simulink model "sldemo_eml_galaxy"  (Simulink 6.0)
settings: Solver=FixedStepDiscrete  StartTime=0.0  StopTime=500  FixedStep=1  RelTol=1e-3
settings Model: Creator=The MathWorks Inc.  LastModifiedBy=batserve  ExtModeAutoUpdateStatusClock=off
settings DebuggingCC: CheckExecutionContextPreStartOutputMsg=on  CheckExecutionContextRuntimeOutputMsg=on

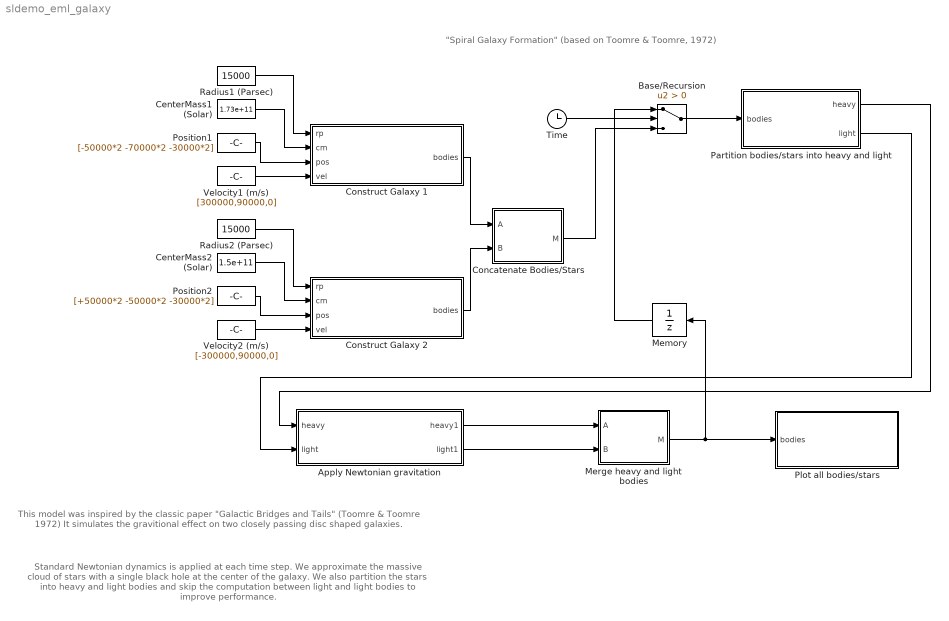
== system sldemo_eml_galaxy ==
  note: "Spiral Galaxy Formation" (based on Toomre & Toomre, 1972)
  note: This model was inspired by the classic paper "Galactic Bridges and Tails" (Toomre & Toomre 1972)
      |  It simulates the gravitional effect on two closely passing disc shaped galaxies.
  note: Standard Newtonian dynamics is applied at each time step. We approximate the massive cloud of stars
      | with a single black hole at the center of the galaxy. We also partition the stars into heavy and light bodies
      | and skip the computation between light and light bodies to improve performance.
  Apply Newtonian gravitation : Stateflow chart  PropExecContextAcrossSSBoundary=on
  Base/Recursion : Switch  Criteria=u2 > Threshold  ZeroCross=off
  CenterMass1 (Solar) : Constant  Value=1.73e+11
  CenterMass2 (Solar) : Constant  Value=1.5e+11
  Concatenate Bodies/Stars : Stateflow chart  PropExecContextAcrossSSBoundary=on
  Construct Galaxy 1 : Stateflow chart  PropExecContextAcrossSSBoundary=on
  Construct Galaxy 2 : Stateflow chart  PropExecContextAcrossSSBoundary=on
  Memory : UnitDelay  Orientation=left  SampleTime=-1
  Merge heavy and light bodies : Stateflow chart  PropExecContextAcrossSSBoundary=on
  Partition bodies/stars into heavy and light : Stateflow chart  PropExecContextAcrossSSBoundary=on
  Plot all bodies/stars : Stateflow chart  PropExecContextAcrossSSBoundary=on
  Position1 : Constant  Value=[-50000*2 -70000*2 -30000*2]
  Position2 : Constant  Value=[+50000*2 -50000*2 -30000*2]
  Radius1 (Parsec) : Constant  Value=15000
  Radius2 (Parsec) : Constant  Value=15000
  Time : Clock
      settings: Decimation=10
  Velocity1 (m/s) : Constant  Value=[300000,90000,0]
  Velocity2 (m/s) : Constant  Value=[-300000,90000,0]
  wires:
  Radius1 (Parsec)/1 -> Construct Galaxy 1/1(rp)
  CenterMass1 (Solar)/1 -> Construct Galaxy 1/2(cm)
  Partition bodies/stars into heavy and light/1(heavy) -> Apply Newtonian gravitation/1(heavy)
  Partition bodies/stars into heavy and light/2(light) -> Apply Newtonian gravitation/2(light)
  Apply Newtonian gravitation/1(heavy1) -> Merge heavy and light bodies/1(A)
  Apply Newtonian gravitation/2(light1) -> Merge heavy and light bodies/2(B)
  Merge heavy and light bodies/1(M) -> Plot all bodies/stars/1(bodies), Memory/1
  Time/1 -> Base/Recursion/2
  Base/Recursion/1 -> Partition bodies/stars into heavy and light/1(bodies)
  Memory/1 -> Base/Recursion/1
  Position1/1 -> Construct Galaxy 1/3(pos)
  Velocity1 (m/s)/1 -> Construct Galaxy 1/4(vel)
  Radius2 (Parsec)/1 -> Construct Galaxy 2/1(rp)
  CenterMass2 (Solar)/1 -> Construct Galaxy 2/2(cm)
  Position2/1 -> Construct Galaxy 2/3(pos)
  Velocity2 (m/s)/1 -> Construct Galaxy 2/4(vel)
  Construct Galaxy 2/1(bodies) -> Concatenate Bodies/Stars/2(B)
  Construct Galaxy 1/1(bodies) -> Concatenate Bodies/Stars/1(A)
  Concatenate Bodies/Stars/1(M) -> Base/Recursion/3

== matlab function Plot all bodies/stars ==
  data: bodies input inherited
function PlotAll(bodies)

persistent fig;
persistent oldPlot;

n = size(bodies,1);

SpeedOfLight = 299792458; % in m/s
YearInSeconds = 365*24*60*60;
LightYear = SpeedOfLight*YearInSeconds;
Parsec = 3.26*LightYear;

if isempty(fig)
    foundFig = findobj('Tag','galaxyScreen');
    if isempty(foundFig)
        fig = figure;
    else
        fig = figure(foundFig);
    end;
    clf(fig);
    set(fig, 'Name', 'Galaxy');
    set(fig, 'DoubleBuffer', 'on', 'Tag', 'galaxyScreen');
    set(fig, 'Renderer', 'painters');
    set(fig, 'Color', 'black');
    hold('on');
    fig_axes = 0; % Required for type inference
    fig_axes = get(fig, 'CurrentAxes');
    init_axes(fig_axes);
    text(-3*30000*Parsec,3*30000*Parsec,0,...
        ['Spiral galaxy formation (based on Toomre, 1972)'...
          char(10),'on close encounters.'],...
        'Color','green','FontSize',14);
end

points_x = zeros(1,n);
points_y = zeros(1,n);
points_z = zeros(1,n);
points_col = zeros(1,n);
for i = 1:n,
    points_x(i) = bodies(i,2);
    points_y(i) = bodies(i,3);
    points_z(i) = bodies(i,4);
    points_col(i) = bodies(i,8);
end

%
% Remove the old plot
%
if isempty(oldPlot)
    oldPlot = 0;
else
    delete(oldPlot);
end

oldPlot = plot3(points_x,points_y,points_z,'w.');
drawnow;

function init_axes(a)
    SpeedOfLight = 299792458; % in m/s
    YearInSeconds = 365*24*60*60;
    LightYear = SpeedOfLight*YearInSeconds;
    Parsec = 3.26*LightYear;
    set(a, 'CameraTarget', [0,0,0] );
    set(a, 'CameraPosition', [0,22000*Parsec*3,18000*Parsec*3]);
    set(a, 'CameraViewAngle', 80 );
    set(a, 'CameraUpVector', [0,1,0]);
    set(a, 'Visible', 'off' ); 
    set(a, 'XLim', [-30000*Parsec*8,30000*Parsec*8]);
    set(a, 'YLim', [-30000*Parsec*8,30000*Parsec*8]);
    set(a, 'ZLim', [-30000*Parsec*8,30000*Parsec*8]);
    set(a, 'DrawMode', 'fast');

== matlab function Construct Galaxy 1 ==
  data: rp input inherited; cm input inherited; bodies output inherited; pos input inherited; vel input inherited
function bodies = ConstructGalaxy(rp,cm,pos,vel)

numberOfBodies = 350;

bodies = ConstructGalaxy0(rp,cm,pos,vel,numberOfBodies);

function bodies = ConstructGalaxy0(rp,cm,pos,vel,n)

SolarMass = 1.9891e+30; % In kg 
G = 6.672E-11; % Nm^2/kg^2 (Gravitational constant)
SpeedOfLight = 299792458; % in m/s
YearInSeconds = 365*24*60*60;
LightYear = SpeedOfLight*YearInSeconds;
Parsec = 3.26*LightYear;

radiusOuter = rp*Parsec;
radiusInner = (rp/3)*Parsec;

% Each star has X,Y,Z,VX,VY,VZ
% X,Y,Z position in certesian coordinates
% VX,VY,VZ velocity in certesian coordinates

cm = cm*SolarMass;

bodies = zeros(n,8);
bodies(1,1) = cm;
bodies(1,2) = pos(1)*Parsec;
bodies(1,3) = pos(2)*Parsec;
bodies(1,4) = pos(3)*Parsec;
bodies(1,5) = vel(1);
bodies(1,6) = vel(2);
bodies(1,7) = vel(3);
bodies(1,8) = 'r';
if n > 1
for i = 2:n,
    m0 = 0;
    m0 = rand();
    m0 = m0*20+4;
    m = m0*SolarMass;
    r0 = 0;
    r0 = rand();
    r = r0*(radiusOuter - radiusInner) + radiusInner;
    arg0 = 0;
    arg0 = rand();
    arg = arg0*2*pi;
    x = r*cos(arg);
    y = r*sin(arg);
    z = 0;
    dx = cos(arg+pi/2);
    dy = sin(arg+pi/2);
    dz = 0;
    % Compute free fall velocity
    v = sqrt(G*cm/r);
    bodies(i,1) = m;
    bodies(i,2) = x+pos(1)*Parsec;
    bodies(i,3) = y+pos(2)*Parsec;
    bodies(i,4) = z+pos(3)*Parsec;
    bodies(i,5) = dx*v+vel(1);
    bodies(i,6) = dy*v+vel(2);
    bodies(i,7) = dz*v+vel(3);
    bodies(i,8) = 'r';
end
end

== matlab function Apply Newtonian gravitation ==
  data: heavy input inherited; heavy1 output inherited; light input inherited; light1 output inherited
function [heavy1,light1] = ApplyGravity(heavy,light)

G = 6.672E-11; % Nm^2/kg^2 (Gravitational constant)

SpeedOfLight = 299792458; % in m/s
YearInSeconds = 365*24*60*60;
LightYear = SpeedOfLight*YearInSeconds;
Parsec = 3.26*LightYear;

timeStep = 2000000*YearInSeconds;

n = size(heavy,1);
nProps = size(heavy,2);

heavy1 = heavy;
light1 = light;

for i = 1:n,
    mi = heavy(i,1);
    if mi == 0
        break;
    end
    xi = heavy(i,2);
    yi = heavy(i,3);
    zi = heavy(i,4);
    ar = [0 0 0];
    for j = 1:n,
        if i ~= j,
            mj = heavy(j,1);
            if mj == 0
                break;
            end
            xj = heavy(j,2);
            yj = heavy(j,3);
            zj = heavy(j,4);
            d = [xj yj zj] - [xi yi zi];
            dr2 = d(1)*d(1)+d(2)*d(2)+d(3)*d(3);
            ar = ar + (d/sqrt(dr2))*((G*mj)/dr2);
        end
    end
    for k = 1:3
        heavy1(i,4+k) = heavy(i,4+k) + ar(k)*timeStep;
    end        
end

for i = 1:n,
    mi = light(i,1);
    if mi == 0
        break;
    end
    xi = light(i,2);
    yi = light(i,3);
    zi = light(i,4);
    ar = [0 0 0];
    for j = 1:n,
        mj = heavy(j,1);
        if mj == 0
            break;
        end
        xj = heavy(j,2);
        yj = heavy(j,3);
        zj = heavy(j,4);
        d = [xj yj zj] - [xi yi zi];
        dr2 = d(1)*d(1)+ d(2)*d(2) + d(3)*d(3);
        ar = ar + (d/sqrt(dr2))*((G*mj)/dr2);
    end
    for k = 1:3
        light1(i,4+k) = light(i,4+k) + ar(k)*timeStep;
    end
end

for i = 1:n
    for k = 1:3
        heavy1(i,k+1) = heavy1(i,k+1) + timeStep*heavy1(i,k+4);
    end
    for k = 1:3
        light1(i,k+1) = light1(i,k+1) + timeStep*light1(i,k+4);
    end
end

== matlab function Partition bodies/stars into heavy and light ==
  data: bodies input inherited; heavy output inherited; light output inherited
function [heavy,light] = Partition(bodies)

SolarMass = 1.9891e+30; % In kg 
Limit = 100*SolarMass;

n = size(bodies,1);
props = size(bodies,2);
heavy = zeros(n,props);
light = zeros(n,props);

lightIndex = 1;
heavyIndex = 1;

for i = 1:n
    m = bodies(i,1);
    if m < Limit
        light(lightIndex,:) = bodies(i,:);
        lightIndex = lightIndex + 1;
    else
        heavy(heavyIndex,:) = bodies(i,:);
        heavyIndex = heavyIndex + 1;
    end
end

== matlab function Merge heavy and light bodies ==
  data: A input inherited; B input inherited; M output inherited
function M = Merge(A,B)

n = size(A,1);
nProps = size(A,2);
M = zeros(n,nProps);
for i = 1:n
    if A(i,1) == 0
        break;
    end
    M(i,:) = A(i,:);
end
n1 = n - i + 1;
for j = 1:n1
    M(j+i-1,:) = B(j,:);
    if B(i,1) == 0
        break
    end
end

== matlab function Construct Galaxy 2 ==
  data: rp input inherited; cm input inherited; bodies output inherited; pos input inherited; vel input inherited
function bodies = ConstructGalaxy(rp,cm,pos,vel)

numberOfBodies = 350;

bodies = ConstructGalaxy0(rp,cm,pos,vel,numberOfBodies);

function bodies = ConstructGalaxy0(rp,cm,pos,vel,n)

SolarMass = 1.9891e+30; % In kg 
G = 6.672E-11; % Nm^2/kg^2 (Gravitational constant)
SpeedOfLight = 299792458; % in m/s
YearInSeconds = 365*24*60*60;
LightYear = SpeedOfLight*YearInSeconds;
Parsec = 3.26*LightYear;

radiusOuter = rp*Parsec;
radiusInner = (rp/3)*Parsec;

% Each star has X,Y,Z,VX,VY,VZ
% X,Y,Z position in certesian coordinates
% VX,VY,VZ velocity in certesian coordinates

cm = cm*SolarMass;

bodies = zeros(n,8);
bodies(1,1) = cm;
bodies(1,2) = pos(1)*Parsec;
bodies(1,3) = pos(2)*Parsec;
bodies(1,4) = pos(3)*Parsec;
bodies(1,5) = vel(1);
bodies(1,6) = vel(2);
bodies(1,7) = vel(3);
bodies(1,8) = 'y';
if n > 1
for i = 2:n,
    m0 = 0;
    m0 = rand();
    m0 = m0*20+4;
    m = m0*SolarMass;
    r0 = 0;
    r0 = rand();
    r = r0*(radiusOuter - radiusInner) + radiusInner;
    arg0 = 0;
    arg0 = rand();
    arg = arg0*2*pi;
    x = r*cos(arg);
    y = r*sin(arg);
    z = 0;
    dx = cos(arg+pi/2);
    dy = sin(arg+pi/2);
    dz = 0;
    % Compute free fall velocity
    v = sqrt(G*cm/r);
    bodies(i,1) = m;
    bodies(i,2) = x+pos(1)*Parsec;
    bodies(i,3) = y+pos(2)*Parsec;
    bodies(i,4) = z+pos(3)*Parsec;
    bodies(i,5) = dx*v+vel(1);
    bodies(i,6) = dy*v+vel(2);
    bodies(i,7) = dz*v+vel(3);
    bodies(i,8) = 'y';
end
end

== matlab function Concatenate Bodies/Stars ==
  data: A input inherited; B input inherited; M output inherited
function M = Concat(A,B)

M = [A; B];
